simulink model "rpi_controller"  (R2024a)
settings: Solver=FixedStepDiscrete  StartTime=0.0  StopTime=60  RelTol=1e-3  EnableMultiTasking=on
undefined symbols (not defined in the file or in its folder): lut_in_model, lut_out_model
libraries: raspberrypiBasiclib x6, raspberrypiAVlib x1, slpidlib x1
settings Model: SimulationMode=external  ExtModeTrigDuration=2  Creator=sjohnson  LastModifiedBy=sjohnson
settings SolverCC: PositivePriorityOrder=on
settings OptimizationCC: EnhancedBackFolding=on  PassReuseOutputArgsThreshold=0  MaxStackSize=64  OptimizeBlockOrder=speed  DifferentSizesBufferReuse=on  OptimizationCustomize=off
settings DebuggingCC: ParameterTunabilityLossMsg=error
settings HardwareCC: ProdBitPerPointer=32  ProdBitPerSizeT=32  ProdBitPerPtrDiffT=32  ProdLargestAtomicInteger=Long  ProdLargestAtomicFloat=Double  ProdWordSize=32  ProdLongLongMode=on  ProdHWDeviceType=ARM Compatible->ARM Cortex  UseEmbeddedCoderFeatures=off  UseSimulinkCoderFeatures=off
settings RTWCC: Description=Embedded Coder  SystemTargetFile=ert.tlc  HardwareBoard=Raspberry Pi  TLCOptions="-aInlineSetEventsForThisBaseRateFcn=TLC_FALSE -aSuppressMultiTaskScheduler=TLC_FALSE  -aRateBasedStepFcn=0"  TemplateMakefile=ert_default_tmf  Toolchain=GNU GCC Embedded Linux  BuildConfiguration=Faster Runs  GPUComputeCapability=3.5
settings CodeAppCC: ForceParamTrailComments=on  OperatorAnnotations=on  MangleLength=10
settings ERTTargetCC: ERTCustomFileBanners=off  SupportContinuousTime=on  SupportNonInlinedSFcns=on  RemoveResetFunc=off  SupportVariableSizeSignals=on  ModelStepFunctionPrototypeControlCompliant=off  ExtModeTransport=2  ExtModeStaticAlloc=on  ExtModeMexFile=ext_xcp  ExtModeIntrfLevel=Level2 - Open

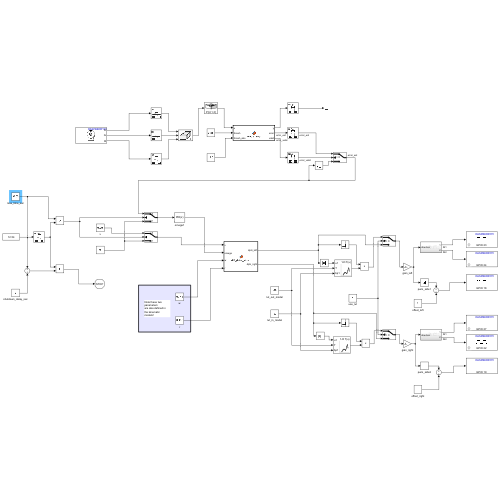
[thumbnail: Simulink's stored preview of the top-level diagram]
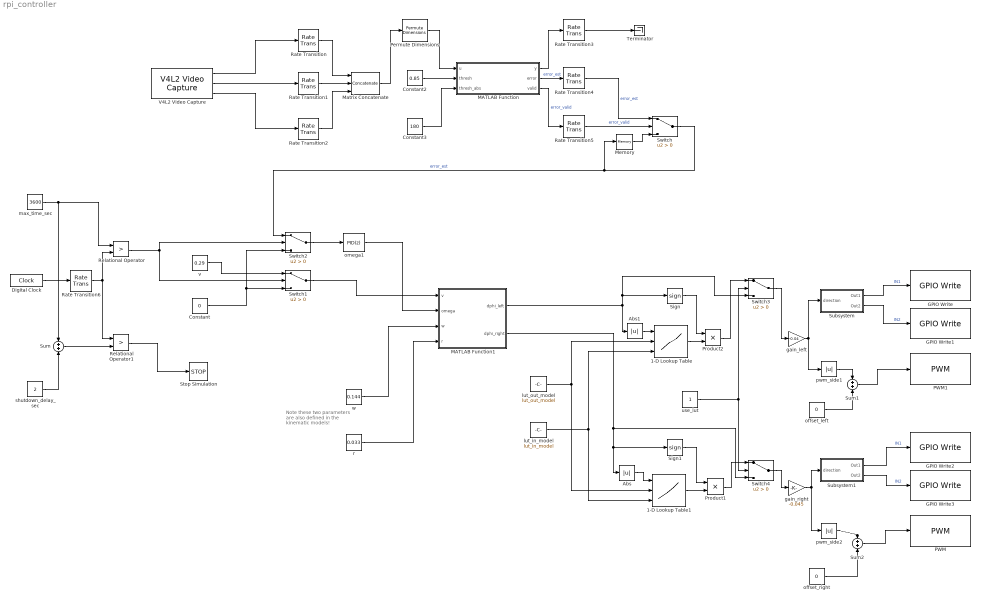
== system rpi_controller ==
  note: Note these two parameters
      | are also defined in the kinematic
      | models!
  1-D Lookup Table : Lookup_n-D  NumberOfTableDimensions=1  BreakpointsForDimension1Source=Input port  BreakpointsForDimension1=[-5:5]  IndexSearchMethod=Linear search  TableSource=Input port  Table=tanh([-5:5])  InterpMethod=Cubic spline  InternalRulePriority=Speed  RndMeth=Simplest
      settings: InputPortMap=u0,p221,p5
  1-D Lookup Table1 : Lookup_n-D  NumberOfTableDimensions=1  BreakpointsForDimension1Source=Input port  BreakpointsForDimension1=[-5:5]  IndexSearchMethod=Linear search  TableSource=Input port  Table=tanh([-5:5])  InterpMethod=Cubic spline  InternalRulePriority=Speed  RndMeth=Simplest
      settings: InputPortMap=u0,p221,p5
  Abs : Abs  SaturateOnIntegerOverflow=off
  Abs1 : Abs  SaturateOnIntegerOverflow=off
  Constant : Constant  Value=0
  Constant2 : Constant  Value=0.85
  Constant3 : Constant  Value=180
  Digital Clock : DigitalClock  SampleTime=1/30
  GPIO Write : raspberrypiBasiclib/GPIO Write  board=Pi 4 Model B  gpio=23  direction=Output  blockPlatform=Raspberry Pi
  GPIO Write1 : raspberrypiBasiclib/GPIO Write  board=Pi 4 Model B  gpio=24  direction=Output  blockPlatform=Raspberry Pi
  GPIO Write2 : raspberrypiBasiclib/GPIO Write  board=Pi 4 Model B  gpio=27  direction=Output  blockPlatform=Raspberry Pi
  GPIO Write3 : raspberrypiBasiclib/GPIO Write  board=Pi 4 Model B  gpio=22  direction=Output  blockPlatform=Raspberry Pi
  MATLAB Function : MATLAB Function  TreatAsAtomicUnit=on
  MATLAB Function1 : MATLAB Function  TreatAsAtomicUnit=on
  Matrix Concatenate : Concatenate  NumInputs=3  Mode=Multidimensional array  ConcatenateDimension=3
  Memory : Memory
  PWM : raspberrypiBasiclib/PWM  board=Pi 4 Model B  Pin_=19  Frequency=40  blockPlatform=Raspberry Pi
  PWM1 : raspberrypiBasiclib/PWM  board=Pi 4 Model B  Pin_=18  Frequency=40  blockPlatform=Raspberry Pi
  Permute Dimensions : PermuteDimensions  Order=[2,1,3]
  Product1 : Product
  Product2 : Product
  Rate Transition{,1..6} (7 alike) : RateTransition
  Relational Operator : RelationalOperator  Operator=>  OutDataTypeStr=boolean  RndMeth=Simplest  InputSameDT=off
  Relational Operator1 : RelationalOperator  Operator=>  OutDataTypeStr=boolean  RndMeth=Simplest  InputSameDT=off
  Sign : Signum
  Sign1 : Signum
  Stop Simulation : Stop
  Subsystem : Subsystem
  Subsystem1 : Subsystem
  Sum : Sum
  Sum1 : Sum
  Sum2 : Sum
  Switch{,1..4} (5 alike) : Switch  Criteria=u2 > Threshold  SaturateOnIntegerOverflow=off  InputSameDT=off
  Terminator : Terminator
  V4L2 Video Capture : raspberrypiAVlib/V4L2 Video Capture  DeviceName=/dev/video0  Resolution=640x480  CustomResolution=[ 320, 240 ]  PixelFormat=RGB  SampleTime=1/30  pixelOrder=planar  simOutput=Colorbars  imSizeSelection=320x240  imSize=[640, 480]  roi=[0, 0, 640, 480]  m_devName='/dev/video0'  blockPlatform=LINUX  HorizontalFlip=off  VerticalFlip=off  Brightness=0.5  Saturation=0.5  Contrast=0.5  Sharpness=0.5  CameraPan=0  CameraTilt=0  CameraZoom=0.5  EnableManualFocus=off  ManualFocus=0.5
  gain_left : Gain  Gain=-0.04
  gain_right : Gain  Gain=-0.045
  lut_in_model : Constant  Value=lut_in_model
  lut_out_model : Constant  Value=lut_out_model
  max_time_sec : Constant  Value=3600
  offset_left : Constant  Value=0
  offset_right : Constant  Value=0
  omega1 : slpidlib/PID Controller  Controller=PID  Form=Parallel  TimeDomain=Discrete-time  UseExternalTs=off  SampleTime=-1  IntegratorMethod=Forward Euler  FilterMethod=Forward Euler  ControllerParametersSource=internal  P=-1.5  I=0  UseKiTs=off  D=0  UseExternalDerivativeSource=off  N=100  UseFilter=on  TunerSelectOption=Transfer Function Based (PID Tuner App)  InitialConditionSource=internal  InitialConditionForIntegrator=0  InitialConditionForFilter=0  DifferentiatorICPrevScaledInput=0  ExternalReset=none  TrackingMode=off  Kt=1  LimitOutput=off  SatLimitsSource=internal  UpperSaturationLimit=inf  LowerSaturationLimit=-inf  LinearizeAsGain=off  AntiWindupMode=none  Kb=1  LimitIntegrator=off  UpperIntegratorSaturationLimit=inf  LowerIntegratorSaturationLimit=-inf  POutMin=[]  POutMax=[]  IOutMin=[]  IOutMax=[]  DOutMin=[]  DOutMax=[]  NOutMin=[]  NOutMax=[]  SumOutMin=[]  SumOutMax=[]  SaturationOutMin=[]  SaturationOutMax=[]  PParamMin=[]  PParamMax=[]  IParamMin=[]  IParamMax=[]  DParamMin=[]  DParamMax=[]  NParamMin=[]  NParamMax=[]  KbParamMin=[]  KbParamMax=[]  KtParamMin=[]  KtParamMax=[]  KbOutMin=[]  KbOutMax=[]  KtOutMin=[]  KtOutMax=[]  IntegratorOutMin=[]  IntegratorOutMax=[]  FilterOutMin=[]  FilterOutMax=[]  SumI1OutMin=[]  SumI1OutMax=[]  SumI2OutMin=[]  SumI2OutMax=[]  SumI3OutMin=[]  SumI3OutMax=[]  SumI4OutMin=[]  SumI4OutMax=[]  SumDOutMin=[]  SumDOutMax=[]  DifferentiatorOutMin=[]  DifferentiatorOutMax=[]  FilterDiffOutCoefMin=[]  FilterDiffOutCoefMax=[]  ReciprocalOutMin=[]  ReciprocalOutMax=[]  SumDenOutMin=[]  SumDenOutMax=[]  SumNumOutMin=[]  SumNumOutMax=[]  DivideOutMin=[]  DivideOutMax=[]  UdiffTsProdOutMin=[]  UdiffTsProdOutMax=[]  NTsProdOutMin=[]  NTsProdOutMax=[]  UintegralTsProdOutMin=[]  UintegralTsProdOutMax=[]  UngainTsProdOutMin=[]  UngainTsProdOutMax=[]  ClampingZeroOutDataTypeStr=Inherit: Inherit via back propagation  ClampingZeroOutMin=[]  ClampingZeroOutMax=[]  FilterDenConstantOutDataTypeStr=Inherit: Inherit via back propagation  FilterDenConstantOutMin=[]  FilterDenConstantOutMax=[]  PCopyOutDataTypeStr=Inherit: Inherit via back propagation  PCopyOutMin=[]  PCopyOutMax=[]  NCopyOutDataTypeStr=Inherit: Inherit via back propagation  NCopyOutMin=[]  NCopyOutMax=[]  IntegratorContinuousStateAttributes=''  IntegratorStateMustResolveToSignalObject=off  IntegratorRTWStateStorageClass=Auto  FilterContinuousStateAttributes=''  FilterStateMustResolveToSignalObject=off  FilterRTWStateStorageClass=Auto  ParallelPVariant=InternalParameters  IdealPVariant=Disabled  IVariant=InternalParameters  DVariant=InternalParameters  IntegratorVariant=Discrete  SatVariant=Disabled  AWVariant=Passthrough  PCopyVariant=Disabled  TRVariant=Disabled  FdbkBlocksVariant=Forward  IdealPFdbkVariant=Disabled  SatFdbkVariant=Disabled  DerivativeFilterVariant=ForwardEulerFilter  NVariant=InternalParameters  NCopyVariant=Disabled  FilterICVariant=InternalICsFilter  IntegratorICVariant=InternalICs  ExternalResetVariant=Disabled  TRSumVariant=Passthrough  SumFdbkVariant=Disabled  SumVariant=Sum_PID  TsampFilterVariant=InternalTs  TsampNgainVariant=Passthrough  TsampIntegralVariant=Disabled_SignalSpec  ExternalSaturationOutDataTypeStr=Inherit: Same as second input  DerivativeSourceVariant=ErrorSignal
      settings: LibrarySourceBlock=simulink/Discrete/Discrete PID Controller
  pwm_side1 : Abs  SaturateOnIntegerOverflow=off
  pwm_side2 : Abs  SaturateOnIntegerOverflow=off
  r : Constant  Value=0.033
  shutdown_delay_sec : Constant  Value=2
  use_lut : Constant
  v : Constant  Value=0.29
  w : Constant  Value=0.144
  wires:
  Constant2/1 -> MATLAB Function/2(thresh)
  Matrix Concatenate/1 -> Permute Dimensions/1
  MATLAB Function/1(y) -> Rate Transition3/1
  Rate Transition2/1 -> Matrix Concatenate/3
  V4L2 Video Capture/2 -> Rate Transition1/1
  Permute Dimensions/1 -> MATLAB Function/1(u)
  V4L2 Video Capture/1 -> Rate Transition/1
  Rate Transition1/1 -> Matrix Concatenate/2
  MATLAB Function/2(error) -> Rate Transition4/1  "error_est"
  MATLAB Function/3(valid) -> Rate Transition5/1  "error_valid"
  V4L2 Video Capture/3 -> Rate Transition2/1
  Constant3/1 -> MATLAB Function/3(thresh_abs)
  Rate Transition/1 -> Matrix Concatenate/1
  r/1 -> MATLAB Function1/4(r)
  w/1 -> MATLAB Function1/3(w)
  v/1 -> Switch1/1
  omega1/1 -> MATLAB Function1/2(omega)
  Switch/1 -> Switch2/1, Memory/1  "error_est"
  Rate Transition5/1 -> Switch/2  "error_valid"
  Rate Transition4/1 -> Switch/1  "error_est"
  Memory/1 -> Switch/3
  Rate Transition3/1 -> Terminator/1
  Digital Clock/1 -> Rate Transition6/1
  Relational Operator/1 -> Switch1/2, Switch2/2
  max_time_sec/1 -> Relational Operator/1, Sum/1
  Rate Transition6/1 -> Relational Operator1/1, Relational Operator/2
  Switch2/1 -> omega1/1
  Switch1/1 -> MATLAB Function1/1(v)
  Constant/1 -> Switch2/3, Switch1/3
  shutdown_delay_sec/1 -> Sum/2
  Sum/1 -> Relational Operator1/2
  Relational Operator1/1 -> Stop Simulation/1
  Abs/1 -> 1-D Lookup Table1/1
  use_lut/1 -> Switch4/2, Switch3/2
  MATLAB Function1/2(dphi_right) -> Switch4/3, Sign1/1, Abs/1
  MATLAB Function1/1(dphi_left) -> Switch3/3, Sign/1, Abs1/1
  Product2/1 -> Switch3/1
  Switch3/1 -> gain_left/1
  1-D Lookup Table/1 -> Product2/2
  lut_out_model/1 -> 1-D Lookup Table1/2, 1-D Lookup Table/2
  Switch4/1 -> gain_right/1
  Product1/1 -> Switch4/1
  Sign1/1 -> Product1/1
  lut_in_model/1 -> 1-D Lookup Table1/3, 1-D Lookup Table/3
  Sign/1 -> Product2/1
  Subsystem/2(Out2) -> GPIO Write1/1  "IN2"
  pwm_side2/1 -> Sum2/1
  Subsystem1/2(Out2) -> GPIO Write3/1  "IN2"
  gain_right/1 -> pwm_side2/1, Subsystem1/1(direction)
  Subsystem1/1(Out1) -> GPIO Write2/1  "IN1"
  Sum1/1 -> PWM1/1
  offset_left/1 -> Sum1/2
  offset_right/1 -> Sum2/2
  Sum2/1 -> PWM/1
  Abs1/1 -> 1-D Lookup Table/1
  Subsystem/1(Out1) -> GPIO Write/1  "IN1"
  pwm_side1/1 -> Sum1/1
  1-D Lookup Table1/1 -> Product1/2
  gain_left/1 -> pwm_side1/1, Subsystem/1(direction)

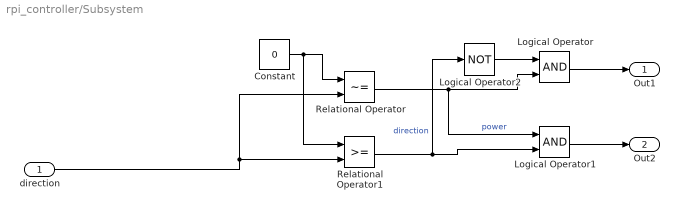
== system rpi_controller/Subsystem ==
  direction : Inport
  Constant : Constant  Value=0
  Logical Operator : Logic  AllPortsSameDT=off  OutDataTypeStr=boolean
  Logical Operator1 : Logic  AllPortsSameDT=off  OutDataTypeStr=boolean
  Logical Operator2 : Logic  Operator=NOT  Inputs=1  AllPortsSameDT=off  OutDataTypeStr=boolean
  Relational Operator : RelationalOperator  Operator=~=  OutDataTypeStr=boolean  RndMeth=Simplest  InputSameDT=off
  Relational Operator1 : RelationalOperator  OutDataTypeStr=boolean  RndMeth=Simplest  InputSameDT=off
  Out1 : Outport
  Out2 : Outport  Port=2
  wires:
  Logical Operator/1 -> Out1/1
  Relational Operator1/1 -> Logical Operator2/1, Logical Operator1/2  "direction"
  Logical Operator1/1 -> Out2/1
  Logical Operator2/1 -> Logical Operator/1
  direction/1 -> Relational Operator/2, Relational Operator1/2
  Constant/1 -> Relational Operator1/1, Relational Operator/1
  Relational Operator/1 -> Logical Operator1/1, Logical Operator/2  "power"

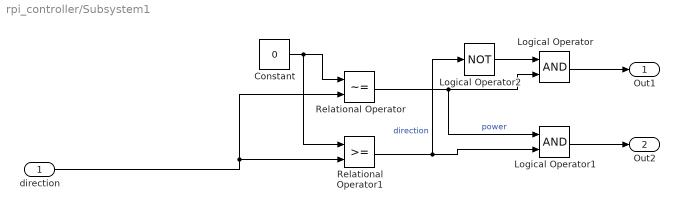
== system rpi_controller/Subsystem1 ==
  direction : Inport
  Constant : Constant  Value=0
  Logical Operator : Logic  AllPortsSameDT=off  OutDataTypeStr=boolean
  Logical Operator1 : Logic  AllPortsSameDT=off  OutDataTypeStr=boolean
  Logical Operator2 : Logic  Operator=NOT  Inputs=1  AllPortsSameDT=off  OutDataTypeStr=boolean
  Relational Operator : RelationalOperator  Operator=~=  OutDataTypeStr=boolean  RndMeth=Simplest  InputSameDT=off
  Relational Operator1 : RelationalOperator  OutDataTypeStr=boolean  RndMeth=Simplest  InputSameDT=off
  Out1 : Outport
  Out2 : Outport  Port=2
  wires:
  Logical Operator/1 -> Out1/1
  Relational Operator1/1 -> Logical Operator2/1, Logical Operator1/2  "direction"
  Logical Operator1/1 -> Out2/1
  Logical Operator2/1 -> Logical Operator/1
  direction/1 -> Relational Operator/2, Relational Operator1/2
  Constant/1 -> Relational Operator1/1, Relational Operator/1
  Relational Operator/1 -> Logical Operator1/1, Logical Operator/2  "power"

== matlab function rpi_controller/MATLAB Function1 ==
  data: v input; dphi_left output; omega input; w input; r input; dphi_right output
function [dphi_left, dphi_right] = diff_drive_xform(v, omega, w, r)

c1 = w/(2*r);
c2 = 2/w;

dphi_left = c1 * ( c2*v - omega );
dphi_right = c1 * ( c2*v + omega );

== matlab function rpi_controller/MATLAB Function ==
  data: u input; y output; error output; valid output; thresh input; thresh_abs input
function [y, error, valid] = image_strip(u, thresh, thresh_abs)
% trim out horizontal slice of image
y = u(325:425, :, :);
dy = double(y);
redness = dy(:,:,1)./vecnorm(dy,1,3) .* dy(:,:,1)>thresh_abs;
y_reduction = max(redness,[],1);
fmin = find(y_reduction>thresh, 1, 'first');
fmax = find(y_reduction>thresh, 1, 'last');
if isempty(fmin) | isempty(fmax)
    valid = 0;
    error = nan;
else
    valid = 1;
    min_value = [find(y_reduction>thresh, 1, 'first')];
    max_value = [find(y_reduction>thresh, 1, 'last')];
    error = ((max_value(1) + min_value(1))/2 - 320)/320;
end
